simulink model "model"  (R2024a)
settings: Solver=ode4  StartTime=0.0  StopTime=6  FixedStep=0.01  RelTol=1e-3
undefined symbols (not defined in the file): a_0, a_1, y0, yy0
settings Model: Creator=TAU  LastModifiedBy=main

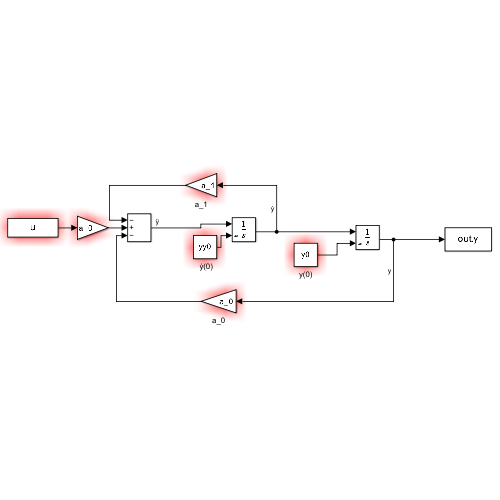
[thumbnail: Simulink's stored preview of the top-level diagram]
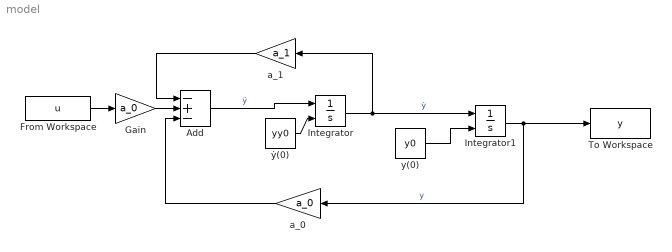
== system model ==
  " ẏ(0)" : Constant  Value=yy0
  Add : Sum  Inputs=-+-
  From Workspace : FromWorkspace  VariableName=u
  Gain : Gain  Gain=a_0
  Integrator : Integrator  InitialConditionSource=external
  Integrator1 : Integrator  InitialConditionSource=external
  To Workspace : ToWorkspace  VariableName=y  SaveFormat=Timeseries  SampleTime=-1
  a_0 : Gain  Gain=a_0
  a_1 : Gain  Gain=a_1
  y(0) : Constant  Value=y0
  wires:
  Integrator/1 -> a_1/1, Integrator1/1  "ẏ"
  Integrator1/1 -> a_0/1, To Workspace/1  "y"
  Add/1 -> Integrator/1  "ÿ"
  " ẏ(0)"/1 -> Integrator/2
  y(0)/1 -> Integrator1/2
  a_1/1 -> Add/1
  a_0/1 -> Add/3
  From Workspace/1 -> Gain/1
  Gain/1 -> Add/2
